simulink model "ex_modeling_data"  (Simulink 10.0)
settings: Solver=VariableStepAuto  StartTime=0.0  StopTime=30  RelTol=1e-3
PreLoadFcn:
  | run(fullfile(matlabroot,'examples','simulink','main',...
  | 'ex_modeling_data_variables.m'))
undefined symbols (not defined in the file): c, k, kdAngle, kdHeight, kiAngle, kiHeight, kpAngle, kpHeight, m, nAngle, nHeight
libraries: simulink x2
settings Model: Creator=The MathWorks, Inc.  LastModifiedBy=bhisma
settings DataIOCC: SaveFormat=Dataset
settings OptimizationCC: LifeSpan=auto
settings DebuggingCC: UnderspecifiedInitializationDetection=Simplified  MergeDetectMultiDrivingBlocksExec=error  PregeneratedLibrarySubsystemCodeDiagnostic=none  SFUnexpectedBacktrackingDiag=error  SFNoUnconditionalDefaultTransitionDiag=error  SFExecutionAtInitializationDiag=warning
settings HardwareCC: ProdBitPerPointer=64  ProdBitPerSizeT=64  ProdBitPerPtrDiffT=64  ProdLargestAtomicFloat=Float  ProdIntDivRoundTo=Zero  ProdEndianess=LittleEndian  ProdWordSize=64  ProdHWDeviceType=Intel->x86-64 (Windows64)
settings ModelReferenceCC: PropagateSignalLabelsOutOfModel=on
settings CodeAppCC: StateflowObjectComments=off
settings GRTTargetCC: TargetLangStandard=C99 (ISO)  CombineOutputUpdateFcns=on  GRTInterface=off
settings ConfigComp: CovMetricSettings=dwe  CovHtmlReporting=off  CovSaveCumulativeToWorkspaceVar=off  CovSaveSingleToWorkspaceVar=off

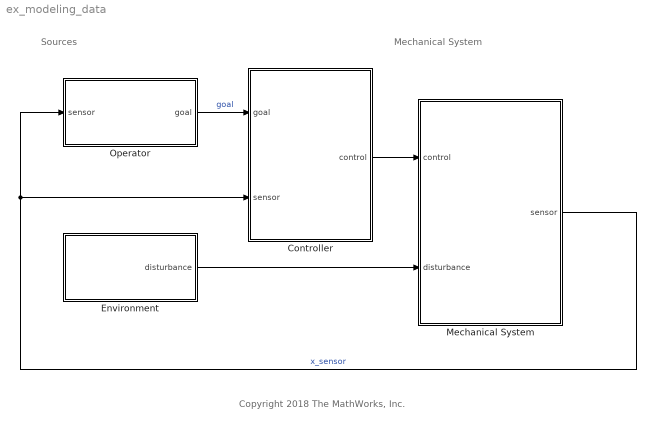
== system ex_modeling_data ==
  note: Mechanical System
  note: Sources
  note: Copyright 2018 The MathWorks, Inc.
  Controller : Subsystem
  Environment : Subsystem
  Mechanical System : Subsystem
  Operator : Subsystem
  wires:
  Operator/1(goal) -> Controller/1(goal)  "goal"
  Controller/1("control ") -> Mechanical System/1(control)
  Mechanical System/1(sensor) -> Controller/2(sensor), Operator/1(sensor)  "x_sensor"
  Environment/1(disturbance) -> Mechanical System/2(disturbance)

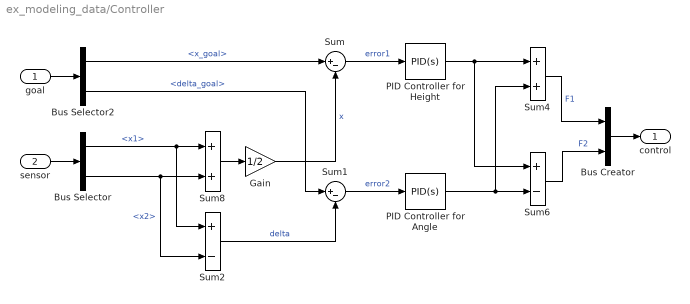
== system ex_modeling_data/Controller ==
  goal : Inport
  sensor : Inport  Port=2
  Bus Creator : BusCreator  Inputs=2
  Bus Selector : BusSelector  OutputSignals=x1,x2
  Bus Selector2 : BusSelector  OutputSignals=x_goal,delta_goal
  Gain : Gain  Gain=1/2
  PID Controller for Angle : simulink/Continuous/PID Controller  Controller=PID  Form=Parallel  TimeDomain=Continuous-time  SampleTime=-1  IntegratorMethod=Forward Euler  FilterMethod=Forward Euler  ControllerParametersSource=internal  P=kpAngle  I=kiAngle  D=kdAngle  UseFilter=on  N=nAngle  TunerSelectOption=Transfer Function Based (PID Tuner App)  InitialConditionSource=internal  InitialConditionForIntegrator=0  InitialConditionForFilter=0  DifferentiatorICPrevScaledInput=0  ExternalReset=none  TrackingMode=off  Kt=1  LimitOutput=off  UpperSaturationLimit=inf  LowerSaturationLimit=-inf  LinearizeAsGain=on  AntiWindupMode=none  Kb=1  POutMin=[]  POutMax=[]  IOutMin=[]  IOutMax=[]  DOutMin=[]  DOutMax=[]  NOutMin=[]  NOutMax=[]  SumOutMin=[]  SumOutMax=[]  SaturationOutMin=[]  SaturationOutMax=[]  PParamMin=[]  PParamMax=[]  IParamMin=[]  IParamMax=[]  DParamMin=[]  DParamMax=[]  NParamMin=[]  NParamMax=[]  KbParamMin=[]  KbParamMax=[]  KtParamMin=[]  KtParamMax=[]  KbOutMin=[]  KbOutMax=[]  KtOutMin=[]  KtOutMax=[]  IntegratorOutMin=[]  IntegratorOutMax=[]  FilterOutMin=[]  FilterOutMax=[]  SumI1OutMin=[]  SumI1OutMax=[]  SumI2OutMin=[]  SumI2OutMax=[]  SumI3OutMin=[]  SumI3OutMax=[]  SumI4OutMin=[]  SumI4OutMax=[]  SumDOutMin=[]  SumDOutMax=[]  DifferentiatorOutMin=[]  DifferentiatorOutMax=[]  FilterDiffOutCoefMin=[]  FilterDiffOutCoefMax=[]  ReciprocalOutMin=[]  ReciprocalOutMax=[]  SumDenOutMin=[]  SumDenOutMax=[]  SumNumOutMin=[]  SumNumOutMax=[]  DivideOutMin=[]  DivideOutMax=[]  IntegratorContinuousStateAttributes=''  IntegratorStateMustResolveToSignalObject=off  IntegratorRTWStateStorageClass=Auto  FilterContinuousStateAttributes=''  FilterStateMustResolveToSignalObject=off  FilterRTWStateStorageClass=Auto  ParallelPVariant=InternalParameters  IdealPVariant=Disabled  IVariant=InternalParameters  DVariant=InternalParameters  IntegratorVariant=Continuous  SatVariant=Disabled  AWVariant=Passthrough  PCopyVariant=Disabled  TRVariant=Disabled  FdbkBlocksVariant=Forward  IdealPFdbkVariant=Disabled  SatFdbkVariant=Disabled  DerivativeFilterVariant=ContFilter  NVariant=InternalParameters  NCopyVariant=Disabled  FilterICVariant=InternalICsFilter  IntegratorICVariant=InternalICs  ExternalResetVariant=Disabled  TRSumVariant=Passthrough  SumFdbkVariant=Disabled  SumVariant=Sum_PID
  PID Controller for Height : simulink/Continuous/PID Controller  Controller=PID  Form=Parallel  TimeDomain=Continuous-time  SampleTime=-1  IntegratorMethod=Forward Euler  FilterMethod=Forward Euler  ControllerParametersSource=internal  P=kpHeight  I=kiHeight  D=kdHeight  UseFilter=on  N=nHeight  TunerSelectOption=Transfer Function Based (PID Tuner App)  InitialConditionSource=internal  InitialConditionForIntegrator=0  InitialConditionForFilter=0  DifferentiatorICPrevScaledInput=0  ExternalReset=none  TrackingMode=off  Kt=1  LimitOutput=off  UpperSaturationLimit=inf  LowerSaturationLimit=-inf  LinearizeAsGain=on  AntiWindupMode=none  Kb=1  POutMin=[]  POutMax=[]  IOutMin=[]  IOutMax=[]  DOutMin=[]  DOutMax=[]  NOutMin=[]  NOutMax=[]  SumOutMin=[]  SumOutMax=[]  SaturationOutMin=[]  SaturationOutMax=[]  PParamMin=[]  PParamMax=[]  IParamMin=[]  IParamMax=[]  DParamMin=[]  DParamMax=[]  NParamMin=[]  NParamMax=[]  KbParamMin=[]  KbParamMax=[]  KtParamMin=[]  KtParamMax=[]  KbOutMin=[]  KbOutMax=[]  KtOutMin=[]  KtOutMax=[]  IntegratorOutMin=[]  IntegratorOutMax=[]  FilterOutMin=[]  FilterOutMax=[]  SumI1OutMin=[]  SumI1OutMax=[]  SumI2OutMin=[]  SumI2OutMax=[]  SumI3OutMin=[]  SumI3OutMax=[]  SumI4OutMin=[]  SumI4OutMax=[]  SumDOutMin=[]  SumDOutMax=[]  DifferentiatorOutMin=[]  DifferentiatorOutMax=[]  FilterDiffOutCoefMin=[]  FilterDiffOutCoefMax=[]  ReciprocalOutMin=[]  ReciprocalOutMax=[]  SumDenOutMin=[]  SumDenOutMax=[]  SumNumOutMin=[]  SumNumOutMax=[]  DivideOutMin=[]  DivideOutMax=[]  IntegratorContinuousStateAttributes=''  IntegratorStateMustResolveToSignalObject=off  IntegratorRTWStateStorageClass=Auto  FilterContinuousStateAttributes=''  FilterStateMustResolveToSignalObject=off  FilterRTWStateStorageClass=Auto  ParallelPVariant=InternalParameters  IdealPVariant=Disabled  IVariant=InternalParameters  DVariant=InternalParameters  IntegratorVariant=Continuous  SatVariant=Disabled  AWVariant=Passthrough  PCopyVariant=Disabled  TRVariant=Disabled  FdbkBlocksVariant=Forward  IdealPFdbkVariant=Disabled  SatFdbkVariant=Disabled  DerivativeFilterVariant=ContFilter  NVariant=InternalParameters  NCopyVariant=Disabled  FilterICVariant=InternalICsFilter  IntegratorICVariant=InternalICs  ExternalResetVariant=Disabled  TRSumVariant=Passthrough  SumFdbkVariant=Disabled  SumVariant=Sum_PID
  Sum : Sum  Inputs=|+-
  Sum1 : Sum  Inputs=|+-
  Sum2 : Sum  Inputs=+-
  Sum4 : Sum
  Sum6 : Sum  Inputs=+-
  Sum8 : Sum
  "control " : Outport  VectorParamsAs1DForOutWhenUnconnected=off
  wires:
  PID Controller for Height/1 -> Sum6/1, Sum4/1
  Sum6/1 -> Bus Creator/2  "F2"
  Sum/1 -> PID Controller for Height/1  "error1"
  PID Controller for Angle/1 -> Sum6/2, Sum4/2
  Sum1/1 -> PID Controller for Angle/1  "error2"
  Sum4/1 -> Bus Creator/1  "F1"
  Sum2/1 -> Sum1/2  "delta"
  Bus Creator/1 -> "control "/1
  Bus Selector/1 -> Sum2/1, Sum8/1  "<x1>"
  Bus Selector/2 -> Sum2/2, Sum8/2  "<x2>"
  sensor/1 -> Bus Selector/1
  Bus Selector2/1 -> Sum/1  "<x_goal>"
  Sum8/1 -> Gain/1
  goal/1 -> Bus Selector2/1
  Bus Selector2/2 -> Sum1/1  "<delta_goal>"
  Gain/1 -> Sum/2  "x"

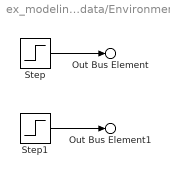
== system ex_modeling_data/Environment ==
  Step : Step  Time=10  After=10  SampleTime=0
  Step1 : Step  Time=20  After=10  SampleTime=0
  Out Bus Element : Outport  VectorParamsAs1DForOutWhenUnconnected=off  PortName=disturbance  Element=F1
  Out Bus Element1 : Outport  VectorParamsAs1DForOutWhenUnconnected=off  PortName=disturbance  Element=F2
  wires:
  Step/1 -> Out Bus Element/1
  Step1/1 -> Out Bus Element1/1

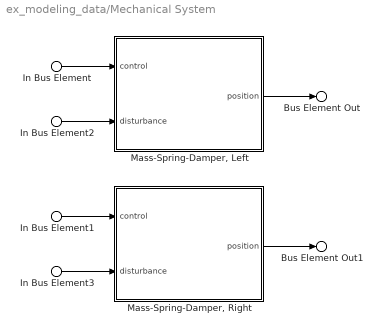
== system ex_modeling_data/Mechanical System ==
  In Bus Element : Inport  PortName=control  Element=F1
  In Bus Element1 : Inport  PortName=control  Element=F2
  In Bus Element2 : Inport  Port=2  PortName=disturbance  Element=F1
  In Bus Element3 : Inport  Port=2  PortName=disturbance  Element=F2
  "Mass-Spring-Damper, Left" : Subsystem
  "Mass-Spring-Damper, Right" : Subsystem
  Bus Element Out : Outport  VectorParamsAs1DForOutWhenUnconnected=off  PortName=sensor  Element=x1
  Bus Element Out1 : Outport  VectorParamsAs1DForOutWhenUnconnected=off  PortName=sensor  Element=x2
  wires:
  In Bus Element/1 -> "Mass-Spring-Damper, Left"/1(control)
  In Bus Element1/1 -> "Mass-Spring-Damper, Right"/1(control)
  In Bus Element2/1 -> "Mass-Spring-Damper, Left"/2(disturbance)
  In Bus Element3/1 -> "Mass-Spring-Damper, Right"/2(disturbance)
  "Mass-Spring-Damper, Left"/1(position) -> Bus Element Out/1
  "Mass-Spring-Damper, Right"/1(position) -> Bus Element Out1/1

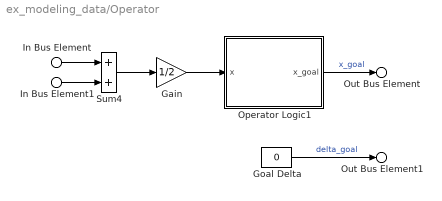
== system ex_modeling_data/Operator ==
  In Bus Element1 : Inport  PortName=sensor  Element=x2
  In Bus Element : Inport  PortName=sensor  Element=x1
  Gain : Gain  Gain=1/2
  Goal Delta : Constant  Value=0
  Operator Logic1 : Stateflow chart  TreatAsAtomicUnit=on
  Sum4 : Sum
  Out Bus Element : Outport  VectorParamsAs1DForOutWhenUnconnected=off  PortName=goal  Element=x_goal
  Out Bus Element1 : Outport  VectorParamsAs1DForOutWhenUnconnected=off  PortName=goal  Element=delta_goal
  wires:
  Operator Logic1/1(x_goal) -> Out Bus Element/1  "x_goal"
  Goal Delta/1 -> Out Bus Element1/1  "delta_goal"
  In Bus Element1/1 -> Sum4/2
  In Bus Element/1 -> Sum4/1
  Gain/1 -> Operator Logic1/1(x)
  Sum4/1 -> Gain/1

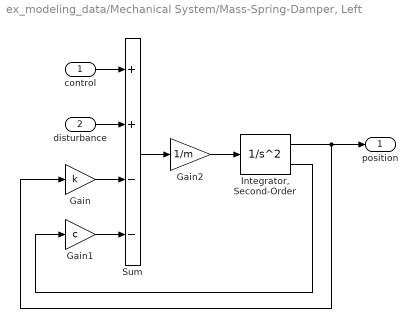
== system ex_modeling_data/Mechanical System/Mass-Spring-Damper, Left ==
  control : Inport
  disturbance : Inport  Port=2
  Gain : Gain  Gain=k
  Gain1 : Gain  Gain=c
  Gain2 : Gain  Gain=1/m
  "Integrator, Second-Order" : SecondOrderIntegrator
  Sum : Sum  Inputs=++--
  position : Outport  VectorParamsAs1DForOutWhenUnconnected=off
  wires:
  Gain/1 -> Sum/3
  control/1 -> Sum/1
  "Integrator, Second-Order"/1 -> position/1, Gain/1
  Gain1/1 -> Sum/4
  "Integrator, Second-Order"/2 -> Gain1/1
  disturbance/1 -> Sum/2
  Gain2/1 -> "Integrator, Second-Order"/1
  Sum/1 -> Gain2/1

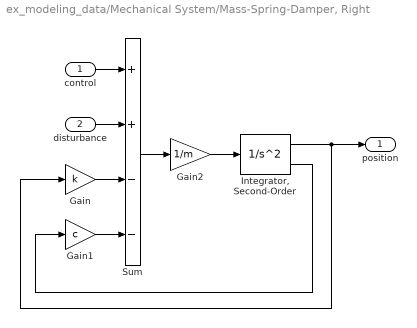
== system ex_modeling_data/Mechanical System/Mass-Spring-Damper, Right ==
  control : Inport
  disturbance : Inport  Port=2
  Gain : Gain  Gain=k
  Gain1 : Gain  Gain=c
  Gain2 : Gain  Gain=1/m
  "Integrator, Second-Order" : SecondOrderIntegrator
  Sum : Sum  Inputs=++--
  position : Outport  VectorParamsAs1DForOutWhenUnconnected=off
  wires:
  Sum/1 -> Gain2/1
  Gain2/1 -> "Integrator, Second-Order"/1
  disturbance/1 -> Sum/2
  "Integrator, Second-Order"/2 -> Gain1/1
  Gain1/1 -> Sum/4
  "Integrator, Second-Order"/1 -> Gain/1, position/1
  control/1 -> Sum/1
  Gain/1 -> Sum/3

== stateflow chart Operator/Operator Logic1 ==
  state wait
    entry: x_goal = 0;
  state FirstOperation
    entry: x_goal = 2;
  state SecondOperation
    entry: x_goal = 1;
  wait -> FirstOperation : after(2,sec)
  FirstOperation -> SecondOperation : [x>2]
  (default) -> wait
  data: x input double; x_goal output double
